simulink model "EngReq_SmkLimCalc1"  (R2016b)
settings: configuration reference "CodeGenConfigSet" (kept outside this file)
values from neighbouring files (symbols this model uses):
  EngReq_bSmkLimCnv_C = Calibration.Parameter    [init_EngReq_SmkLimCalc.m]    (also in init_EngReq_SmkLimCalc_SIL.m = Simulink.Parameter)
  EngReq_bSmkLimIntkP_C = Calibration.Parameter    [init_EngReq_SmkLimCalc.m]    (also in init_EngReq_SmkLimCalc_SIL.m = Simulink.Parameter)
  EngReq_facAFSFlt_C = Calibration.Parameter    [init_EngReq_SmkLimCalc.m]    (also in init_EngReq_SmkLimCalc_SIL.m = Simulink.Parameter)
  EngReq_nSlpLimMin_C = Calibration.Parameter    [init_EngReq_SmkLimCalc.m]    (also in init_EngReq_SmkLimCalc_SIL.m = Simulink.Parameter)
  EngReq_SlpLimNeg_C = Calibration.Parameter    [init_EngReq_SmkLimCalc.m]    (also in init_EngReq_SmkLimCalc_SIL.m = Simulink.Parameter)
  EngReq_SlpLimPos_C = Calibration.Parameter    [init_EngReq_SmkLimCalc.m]    (also in init_EngReq_SmkLimCalc_SIL.m = Simulink.Parameter)
  SmkLim_facSmkATSCor_CUR = Calibration.Parameter    [init_EngReq_SmkLimCalc.m]    (also in init_EngReq_SmkLimCalc_SIL.m = Simulink.Parameter)
  SmkLim_facSmkATSCor_CURX = Calibration.Parameter    [init_EngReq_SmkLimCalc.m]    (also in init_EngReq_SmkLimCalc_SIL.m = Simulink.Parameter)
  SmkLim_facSmkEnvPCor_CUR = Calibration.Parameter    [init_EngReq_SmkLimCalc.m]    (also in init_EngReq_SmkLimCalc_SIL.m = Simulink.Parameter)
  SmkLim_facSmkEnvPCor_CURX = Calibration.Parameter    [init_EngReq_SmkLimCalc.m]    (also in init_EngReq_SmkLimCalc_SIL.m = Simulink.Parameter)
  SmkLim_trqLimSmk_MAP = Calibration.Parameter    [init_EngReq_SmkLimCalc.m]    (also in init_EngReq_SmkLimCalc_SIL.m = Simulink.Parameter)
  SmkLim_trqLimSmk_MAPX = Calibration.Parameter    [init_EngReq_SmkLimCalc.m]    (also in init_EngReq_SmkLimCalc_SIL.m = Simulink.Parameter)
  SmkLim_trqLimSmk_MAPY = Calibration.Parameter    [init_EngReq_SmkLimCalc.m]    (also in init_EngReq_SmkLimCalc_SIL.m = Simulink.Parameter)
  SmkLim_trqLimSmkAFS_MAP = Calibration.Parameter    [init_EngReq_SmkLimCalc.m]    (also in init_EngReq_SmkLimCalc_SIL.m = Simulink.Parameter)
  SmkLim_trqLimSmkAFS_MAPX = Calibration.Parameter    [init_EngReq_SmkLimCalc.m]    (also in init_EngReq_SmkLimCalc_SIL.m = Simulink.Parameter)
  SmkLim_trqLimSmkAFS_MAPY = Calibration.Parameter    [init_EngReq_SmkLimCalc.m]    (also in init_EngReq_SmkLimCalc_SIL.m = Simulink.Parameter)
  SmkLim_trqLimSmkAFSEnvPCor_MAP = Calibration.Parameter    [init_EngReq_SmkLimCalc.m]    (also in init_EngReq_SmkLimCalc_SIL.m = Simulink.Parameter)
  SmkLim_trqLimSmkAFSEnvPCor_MAPX = Calibration.Parameter    [init_EngReq_SmkLimCalc.m]    (also in init_EngReq_SmkLimCalc_SIL.m = Simulink.Parameter)
  SmkLim_trqLimSmkAFSEnvPCor_MAPY = Calibration.Parameter    [init_EngReq_SmkLimCalc.m]    (also in init_EngReq_SmkLimCalc_SIL.m = Simulink.Parameter)
undefined symbols (not defined in the file or in its folder): CEngDsT_tTransf_CURX, EngReq_SmkLimCalc_DT
libraries: CXLib x4
settings Model: Creator=Administrator  LastModifiedBy=xuxingpei
settings ConfigSetRef: SourceLocation=Base Workspace

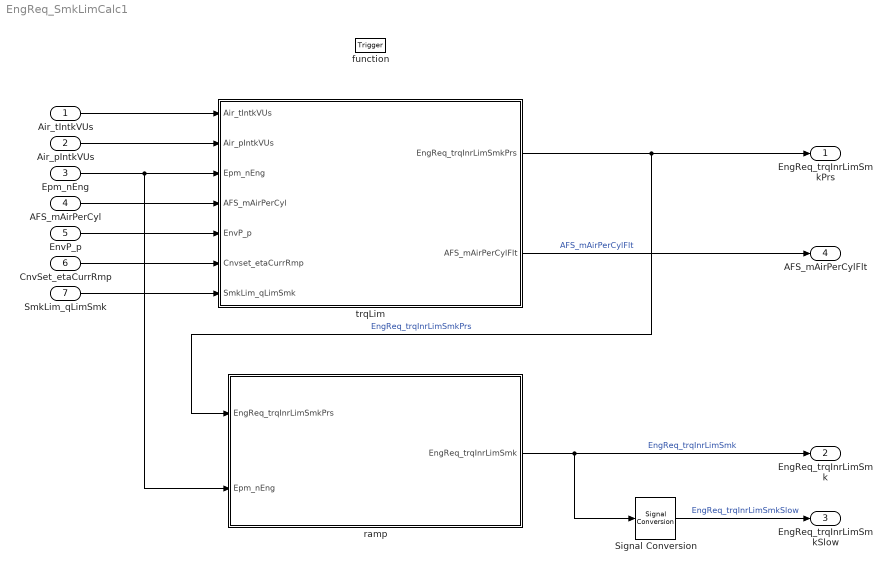
== system EngReq_SmkLimCalc1 ==
  Air_tIntkVUs : Inport  Tag=deg  Description=Intake air temperature upstream of the inlet valve  OutMin=-200  OutMax=200  OutDataTypeStr=Temp_deg
  Air_pIntkVUs : Inport  Tag=kPa  Description=Intake valve upstream pressure  Port=2  OutMin=0  OutMax=1200  OutDataTypeStr=AirPressure_kPa
  Epm_nEng : Inport  Tag=rpm  Description=Engine speed  Port=3  OutMin=0  OutMax=6000  OutDataTypeStr=EngSpeed_rpm
  AFS_mAirPerCyl : Inport  Tag=mg/hub  Description=Air mass per cylinder  Port=4  OutMin=0  OutMax=16383  OutDataTypeStr=AirMass_mg_hub
  EnvP_p : Inport  Tag=kPa  Description=Barometric pressure  Port=5  OutMin=0  OutMax=3276  OutDataTypeStr=AirPressure_kPa
  CnvSet_etaCurrRmp : Inport  Tag=Nm/(mg/hub)  Description=Conversion efficiency corresponding to CnvSet_qSet  Port=6  OutMin=-255  OutMax=255  OutDataTypeStr=TrqEta_Nm_mg_hub
  SmkLim_qLimSmk : Inport  Tag=mg/hub  Description=Smoke limitation quantity in current operation mode  Port=7  OutMin=-319  OutMax=319  OutDataTypeStr=FuelMass_mg_hub
  function : TriggerPort  TriggerType=function-call  VariantControl=Variant
  Signal Conversion : SignalConversion  OverrideOpt=off
  ramp : Subsystem
  trqLim : Subsystem
  EngReq_trqInrLimSmkPrs : Outport  Tag=Nm  Description=Resulting limiting torque smoke limit current operation mode  OutMin=-3276.8  OutMax=3276.7  OutDataTypeStr=Trq_Nm
  EngReq_trqInrLimSmk : Outport  Tag=Nm  Description=Limiting torque smoke limit  Port=2  OutMin=-3276.8  OutMax=3276.7  OutDataTypeStr=Trq_Nm
  EngReq_trqInrLimSmkSlow : Outport  Tag=Nm  Description=Limiting torque smoke limit of slow path  Port=3  OutMin=-3276.8  OutMax=3276.7  OutDataTypeStr=Trq_Nm
  AFS_mAirPerCylFlt : Outport  Tag=mg/hub  Description=filtered Air mass per cylinder  Port=4  OutMin=0  OutMax=16383  OutDataTypeStr=AirMass_mg_hub
  wires:
  Signal Conversion/1 -> EngReq_trqInrLimSmkSlow/1  "EngReq_trqInrLimSmkSlow"
  ramp/1(EngReq_trqInrLimSmk) -> Signal Conversion/1, EngReq_trqInrLimSmk/1  "EngReq_trqInrLimSmk"
  trqLim/1(EngReq_trqInrLimSmkPrs) -> ramp/1(EngReq_trqInrLimSmkPrs), EngReq_trqInrLimSmkPrs/1  "EngReq_trqInrLimSmkPrs"
  Air_tIntkVUs/1 -> trqLim/1(Air_tIntkVUs)
  Air_pIntkVUs/1 -> trqLim/2(Air_pIntkVUs)
  Epm_nEng/1 -> ramp/2(Epm_nEng), trqLim/3(Epm_nEng)
  AFS_mAirPerCyl/1 -> trqLim/4(AFS_mAirPerCyl)
  EnvP_p/1 -> trqLim/5(EnvP_p)
  CnvSet_etaCurrRmp/1 -> trqLim/6(Cnvset_etaCurrRmp)
  SmkLim_qLimSmk/1 -> trqLim/7(SmkLim_qLimSmk)
  trqLim/2(AFS_mAirPerCylFlt) -> AFS_mAirPerCylFlt/1  "AFS_mAirPerCylFlt"

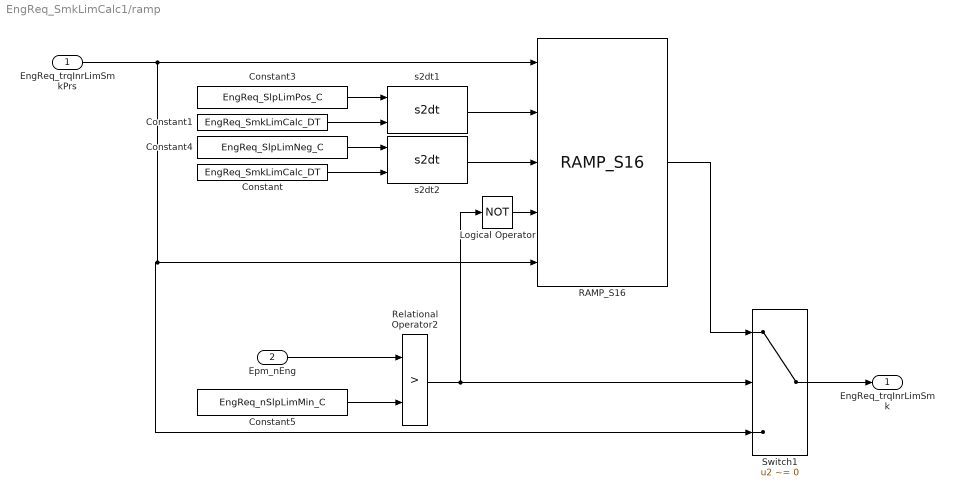
== system EngReq_SmkLimCalc1/ramp ==
  EngReq_trqInrLimSmkPrs : Inport
  Epm_nEng : Inport  Port=2
  Constant : Constant  Value=EngReq_SmkLimCalc_DT
  Constant1 : Constant  Value=EngReq_SmkLimCalc_DT
  Constant3 : Constant  Value=EngReq_SlpLimPos_C
  Constant4 : Constant  Value=EngReq_SlpLimNeg_C
  Constant5 : Constant  Value=EngReq_nSlpLimMin_C
  Logical Operator : Logic  Operator=NOT  AllPortsSameDT=off  OutDataTypeStr=boolean
  RAMP_S16 : CXLib/RAMP_S16
  Relational Operator2 : RelationalOperator  Operator=>  OutDataTypeStr=boolean  RndMeth=Nearest  InputSameDT=on
  Switch1 : Switch  Criteria=u2 ~= 0  SaturateOnIntegerOverflow=on  InputSameDT=on
  s2dt1 : CXLib/s2dt
  s2dt2 : CXLib/s2dt
  EngReq_trqInrLimSmk : Outport
  wires:
  Epm_nEng/1 -> Relational Operator2/1
  Switch1/1 -> EngReq_trqInrLimSmk/1
  Constant/1 -> s2dt2/2
  Constant1/1 -> s2dt1/2
  s2dt2/1 -> RAMP_S16/3
  s2dt1/1 -> RAMP_S16/2
  Constant4/1 -> s2dt2/1
  RAMP_S16/1 -> Switch1/1
  Constant3/1 -> s2dt1/1
  Constant5/1 -> Relational Operator2/2
  Logical Operator/1 -> RAMP_S16/4
  Relational Operator2/1 -> Switch1/2, Logical Operator/1
  EngReq_trqInrLimSmkPrs/1 -> Switch1/3, RAMP_S16/5, RAMP_S16/1

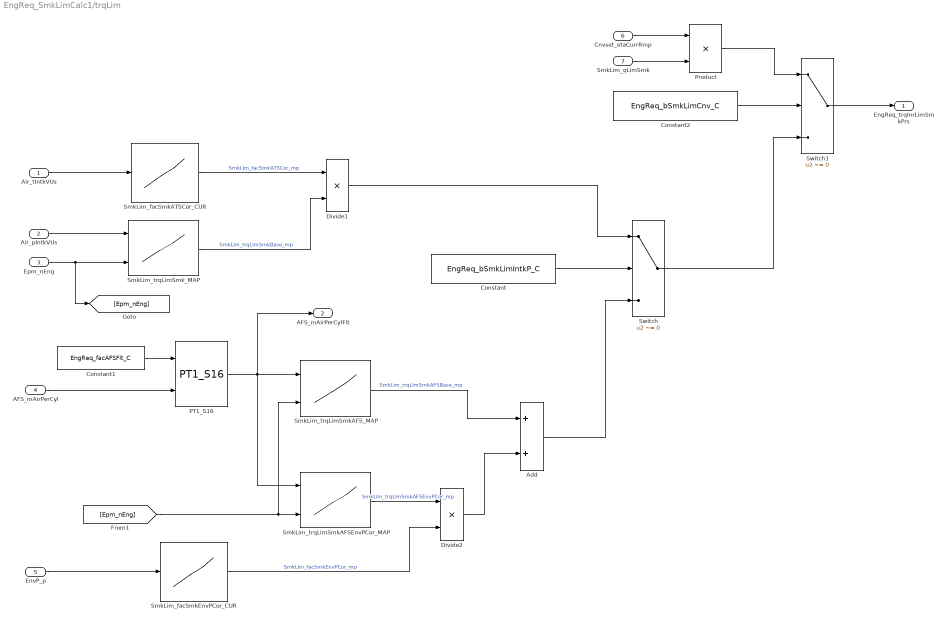
== system EngReq_SmkLimCalc1/trqLim ==
  Air_tIntkVUs : Inport
  Air_pIntkVUs : Inport  Port=2
  Epm_nEng : Inport  Port=3
  AFS_mAirPerCyl : Inport  Port=4
  EnvP_p : Inport  Port=5
  Cnvset_etaCurrRmp : Inport  Tag=Nm/(mg/hub)  Description=Conversion efficiency corresponding to CnvSet_qSet  Port=6  OutMin=-255  OutMax=255  OutDataTypeStr=TrqEta_Nm_mg_hub
  SmkLim_qLimSmk : Inport  Tag=mg/hub  Description=Smoke limitation quantity in current operation mode  Port=7  OutMin=-319  OutMax=319  OutDataTypeStr=FuelMass_mg_hub
  Add : Sum  SaturateOnIntegerOverflow=on  InputSameDT=on  OutDataTypeStr=Inherit: Same as first input
  Constant : Constant  Value=EngReq_bSmkLimIntkP_C
  Constant1 : Constant  Value=EngReq_facAFSFlt_C
  Constant2 : Constant  Value=EngReq_bSmkLimCnv_C
  Divide1 : Product  RequirementInfo={'other' 'HPUn_requirements.docx' '@Simulink_requirement_item_16' 'true' '高压油泵供油量计算' '' } %GIDa_1c05e920_6e57_4613_8bab_1a6d755dd43c  Inputs=**  OutDataTypeStr=Inherit: Inherit via back propagation  RndMeth=Round  SaturateOnIntegerOverflow=on
  Divide2 : Product  RequirementInfo={'other' 'HPUn_requirements.docx' '@Simulink_requirement_item_16' 'true' '高压油泵供油量计算' '' } %GIDa_bfad487e_9857_4251_84d2_3c258dcb33ee  Inputs=**  OutDataTypeStr=Inherit: Inherit via back propagation  RndMeth=Round  SaturateOnIntegerOverflow=on
  PT1_S16 : CXLib/PT1_S16
  Product : Product  OutDataTypeStr=Inherit: Inherit via back propagation  SaturateOnIntegerOverflow=on
  SmkLim_facSmkATSCor_CUR : Lookup_n-D  RequirementInfo={} %GIDa_5f365659_6d96_473e_aa6f_f7b9d531a6f8  DialogController=Simulink.DDGSource  NumberOfTableDimensions=1  BreakpointsForDimension1=SmkLim_facSmkATSCor_CURX  BreakpointsForDimension2=CEngDsT_tTransf_CURX  IndexSearchMethod=Linear search  BeginIndexSearchUsingPreviousIndexResult=on  Table=SmkLim_facSmkATSCor_CUR  ExtrapMethod=Clip  UseLastTableValue=on  InternalRulePriority=Speed  OutDataTypeStr=Inherit: Inherit via back propagation  SaturateOnIntegerOverflow=on
  SmkLim_facSmkEnvPCor_CUR : Lookup_n-D  RequirementInfo={} %GIDa_6b75c835_3f30_46ab_a31a_deeddaf6a614  DialogController=Simulink.DDGSource  NumberOfTableDimensions=1  BreakpointsForDimension1=SmkLim_facSmkEnvPCor_CURX  BreakpointsForDimension2=CEngDsT_tTransf_CURX  BreakpointsForDimension1DataTypeStr=Inherit: Inherit from 'Breakpoint data'  IndexSearchMethod=Linear search  BeginIndexSearchUsingPreviousIndexResult=on  Table=SmkLim_facSmkEnvPCor_CUR  TableDataTypeStr=Inherit: Inherit from 'Table data'  ExtrapMethod=Clip  UseLastTableValue=on  InternalRulePriority=Speed  OutDataTypeStr=Inherit: Inherit from 'Table data'  SaturateOnIntegerOverflow=on
  SmkLim_trqLimSmkAFSEnvPCor_MAP : Lookup_n-D  BreakpointsForDimension1=SmkLim_trqLimSmkAFSEnvPCor_MAPY  BreakpointsForDimension2=SmkLim_trqLimSmkAFSEnvPCor_MAPX  IndexSearchMethod=Linear search  BeginIndexSearchUsingPreviousIndexResult=on  Table=SmkLim_trqLimSmkAFSEnvPCor_MAP  ExtrapMethod=Clip  UseLastTableValue=on  InternalRulePriority=Speed  OutDataTypeStr=Inherit: Inherit via back propagation  RndMeth=Simplest  SaturateOnIntegerOverflow=on
  SmkLim_trqLimSmkAFS_MAP : Lookup_n-D  BreakpointsForDimension1=SmkLim_trqLimSmkAFS_MAPY  BreakpointsForDimension2=SmkLim_trqLimSmkAFS_MAPX  IndexSearchMethod=Linear search  BeginIndexSearchUsingPreviousIndexResult=on  Table=SmkLim_trqLimSmkAFS_MAP  ExtrapMethod=Clip  UseLastTableValue=on  InternalRulePriority=Speed  OutDataTypeStr=Inherit: Inherit via back propagation  RndMeth=Simplest  SaturateOnIntegerOverflow=on
  SmkLim_trqLimSmk_MAP : Lookup_n-D  BreakpointsForDimension1=SmkLim_trqLimSmk_MAPY  BreakpointsForDimension2=SmkLim_trqLimSmk_MAPX  IndexSearchMethod=Linear search  BeginIndexSearchUsingPreviousIndexResult=on  Table=SmkLim_trqLimSmk_MAP  ExtrapMethod=Clip  UseLastTableValue=on  InternalRulePriority=Speed  OutDataTypeStr=Inherit: Inherit via back propagation  RndMeth=Simplest  SaturateOnIntegerOverflow=on
  Switch : Switch  Criteria=u2 ~= 0  InputSameDT=on
  Switch1 : Switch  Criteria=u2 ~= 0  InputSameDT=on
  EngReq_trqInrLimSmkPrs : Outport
  AFS_mAirPerCylFlt : Outport  Tag=mg/hub  Description=filtered Air mass per cylinder  Port=2  OutMin=0  OutMax=16383  OutDataTypeStr=AirMass_mg_hub
  wires:
  [Epm_nEng] -> SmkLim_trqLimSmkAFS_MAP/2, SmkLim_trqLimSmkAFSEnvPCor_MAP/2
  Epm_nEng/1 -> [Epm_nEng], SmkLim_trqLimSmk_MAP/2
  SmkLim_trqLimSmk_MAP/1 -> Divide1/2  "SmkLim_trqLimSmkBase_mp"
  Air_tIntkVUs/1 -> SmkLim_facSmkATSCor_CUR/1
  Air_pIntkVUs/1 -> SmkLim_trqLimSmk_MAP/1
  SmkLim_facSmkATSCor_CUR/1 -> Divide1/1  "SmkLim_facSmkATSCor_mp"
  PT1_S16/1 -> AFS_mAirPerCylFlt/1, SmkLim_trqLimSmkAFSEnvPCor_MAP/1, SmkLim_trqLimSmkAFS_MAP/1
  AFS_mAirPerCyl/1 -> PT1_S16/2
  Add/1 -> Switch/3
  Divide1/1 -> Switch/1
  SmkLim_trqLimSmkAFS_MAP/1 -> Add/1  "SmkLim_trqLimSmkAFSBase_mp"
  Constant1/1 -> PT1_S16/1
  SmkLim_trqLimSmkAFSEnvPCor_MAP/1 -> Divide2/1  "SmkLim_trqLimSmkAFSEnvPCor_mp"
  EnvP_p/1 -> SmkLim_facSmkEnvPCor_CUR/1
  SmkLim_facSmkEnvPCor_CUR/1 -> Divide2/2  "SmkLim_facSmkEnvPCor_mp"
  Divide2/1 -> Add/2
  Constant/1 -> Switch/2
  Switch1/1 -> EngReq_trqInrLimSmkPrs/1
  Switch/1 -> Switch1/3
  Constant2/1 -> Switch1/2
  Cnvset_etaCurrRmp/1 -> Product/1
  SmkLim_qLimSmk/1 -> Product/2
  Product/1 -> Switch1/1
